simulink model "Quad23"  (R2019a)
settings: Solver=ode4  StartTime=0.0  StopTime=23.06  FixedStep=Ts  RelTol=1e-3
values from neighbouring files (symbols this model uses):
  Am = A-B*K_PP    [ALTITUDE_PLUS_ATTITUDE_CONTROL.m]    (also in ALTITUDE_PLUS_ATTITUDE_CONTROL2.m; ALTITUDE_PLUS_ATTITUDE_CONTROL23.m)
  ATTITUDE0 = 1/60*ones(3,1)    [SETUP.m]    (also in SETUP2.m; SETUP23.m)
  Bm = B    [ALTITUDE_PLUS_ATTITUDE_CONTROL.m]    (also in ALTITUDE_PLUS_ATTITUDE_CONTROL2.m; ALTITUDE_PLUS_ATTITUDE_CONTROL23.m)
  Bum = [1 0 0 ... (first row only)    [ALTITUDE_PLUS_ATTITUDE_CONTROL.m]    (also in ALTITUDE_PLUS_ATTITUDE_CONTROL2.m; ALTITUDE_PLUS_ATTITUDE_CONTROL23.m)
  C = [1 0 0 0 0 0 0 ... (first row only)    [ALTITUDE_PLUS_ATTITUDE_CONTROL.m]    (also in ALTITUDE_PLUS_ATTITUDE_CONTROL2.m; ALTITUDE_PLUS_ATTITUDE_CONTROL23.m; LINEARIZZA_ESTRAI.m = [1 0 0 0 0 0 0 0 0 0 0 0)
  D = 1/s    [ALTITUDE_PLUS_ATTITUDE_CONTROL.m]    (also in ALTITUDE_PLUS_ATTITUDE_CONTROL2.m; ALTITUDE_PLUS_ATTITUDE_CONTROL23.m; LINEARIZZA_ESTRAI.m = [0 0 0 0)
  DEN_TF_eta2m_11 = cell2mat(TF_eta2m.Denominator(1,1))    [ALTITUDE_PLUS_ATTITUDE_CONTROL.m]    (also in ALTITUDE_PLUS_ATTITUDE_CONTROL2.m; ALTITUDE_PLUS_ATTITUDE_CONTROL23.m)
  DEN_TF_eta2m_12 = cell2mat(TF_eta2m.Denominator(1,2))    [ALTITUDE_PLUS_ATTITUDE_CONTROL.m]    (also in ALTITUDE_PLUS_ATTITUDE_CONTROL2.m; ALTITUDE_PLUS_ATTITUDE_CONTROL23.m)
  DEN_TF_eta2m_13 = cell2mat(TF_eta2m.Denominator(1,3))    [ALTITUDE_PLUS_ATTITUDE_CONTROL.m]    (also in ALTITUDE_PLUS_ATTITUDE_CONTROL2.m; ALTITUDE_PLUS_ATTITUDE_CONTROL23.m)
  DEN_TF_eta2m_21 = cell2mat(TF_eta2m.Denominator(2,1))    [ALTITUDE_PLUS_ATTITUDE_CONTROL.m]    (also in ALTITUDE_PLUS_ATTITUDE_CONTROL2.m; ALTITUDE_PLUS_ATTITUDE_CONTROL23.m)
  DEN_TF_eta2m_22 = cell2mat(TF_eta2m.Denominator(2,2))    [ALTITUDE_PLUS_ATTITUDE_CONTROL.m]    (also in ALTITUDE_PLUS_ATTITUDE_CONTROL2.m; ALTITUDE_PLUS_ATTITUDE_CONTROL23.m)
  DEN_TF_eta2m_23 = cell2mat(TF_eta2m.Denominator(2,3))    [ALTITUDE_PLUS_ATTITUDE_CONTROL.m]    (also in ALTITUDE_PLUS_ATTITUDE_CONTROL2.m; ALTITUDE_PLUS_ATTITUDE_CONTROL23.m)
  DEN_TF_eta2m_31 = cell2mat(TF_eta2m.Denominator(3,1))    [ALTITUDE_PLUS_ATTITUDE_CONTROL.m]    (also in ALTITUDE_PLUS_ATTITUDE_CONTROL2.m; ALTITUDE_PLUS_ATTITUDE_CONTROL23.m)
  DEN_TF_eta2m_32 = cell2mat(TF_eta2m.Denominator(3,2))    [ALTITUDE_PLUS_ATTITUDE_CONTROL.m]    (also in ALTITUDE_PLUS_ATTITUDE_CONTROL2.m; ALTITUDE_PLUS_ATTITUDE_CONTROL23.m)
  DEN_TF_eta2m_33 = cell2mat(TF_eta2m.Denominator(3,3))    [ALTITUDE_PLUS_ATTITUDE_CONTROL.m]    (also in ALTITUDE_PLUS_ATTITUDE_CONTROL2.m; ALTITUDE_PLUS_ATTITUDE_CONTROL23.m)
  DEN_TF_eta2m_41 = cell2mat(TF_eta2m.Denominator(4,1))    [ALTITUDE_PLUS_ATTITUDE_CONTROL.m]    (also in ALTITUDE_PLUS_ATTITUDE_CONTROL2.m; ALTITUDE_PLUS_ATTITUDE_CONTROL23.m)
  DEN_TF_eta2m_42 = cell2mat(TF_eta2m.Denominator(4,2))    [ALTITUDE_PLUS_ATTITUDE_CONTROL.m]    (also in ALTITUDE_PLUS_ATTITUDE_CONTROL2.m; ALTITUDE_PLUS_ATTITUDE_CONTROL23.m)
  DEN_TF_eta2m_43 = cell2mat(TF_eta2m.Denominator(4,3))    [ALTITUDE_PLUS_ATTITUDE_CONTROL.m]    (also in ALTITUDE_PLUS_ATTITUDE_CONTROL2.m; ALTITUDE_PLUS_ATTITUDE_CONTROL23.m)
  denD = cell2mat(D.Denominator)    [ALTITUDE_PLUS_ATTITUDE_CONTROL.m]    (also in ALTITUDE_PLUS_ATTITUDE_CONTROL2.m; ALTITUDE_PLUS_ATTITUDE_CONTROL23.m)
  g = 9.81    [SETUP.m]    (also in SETUP2.m; SETUP23.m)
  inertia = diag([Ix,Iy,Iz])    [ALTITUDE_PLUS_ATTITUDE_CONTROL.m]    (also in ALTITUDE_PLUS_ATTITUDE_CONTROL2.m; ALTITUDE_PLUS_ATTITUDE_CONTROL23.m; SETUP.m; SETUP2.m)
  K = 180*eye(m_)    [ALTITUDE_PLUS_ATTITUDE_CONTROL.m]    (also in ALTITUDE_PLUS_ATTITUDE_CONTROL2.m; ALTITUDE_PLUS_ATTITUDE_CONTROL23.m)
  K_PP = place(A,B,pole_TARGET)    [ALTITUDE_PLUS_ATTITUDE_CONTROL.m]    (also in ALTITUDE_PLUS_ATTITUDE_CONTROL2.m; ALTITUDE_PLUS_ATTITUDE_CONTROL23.m)
  Kg = -(C*Am^-1*Bm)^-1    [ALTITUDE_PLUS_ATTITUDE_CONTROL.m]    (also in ALTITUDE_PLUS_ATTITUDE_CONTROL2.m; ALTITUDE_PLUS_ATTITUDE_CONTROL23.m)
  Ksp = -eye(size(Am))*0    [ALTITUDE_PLUS_ATTITUDE_CONTROL.m]    (also in ALTITUDE_PLUS_ATTITUDE_CONTROL2.m; ALTITUDE_PLUS_ATTITUDE_CONTROL23.m)
  LAMBDA = [Kf Kf Kf Kf ... (first row only)    [SETUP.m]    (also in SETUP2.m; SETUP23.m)
  LAMBDA_true = LAMBDA +0.005*randn(size(LAMBDA))*0    [ALTITUDE_PLUS_ATTITUDE_CONTROL.m]    (also in ALTITUDE_PLUS_ATTITUDE_CONTROL2.m; ALTITUDE_PLUS_ATTITUDE_CONTROL23.m)
  m = 2.356    [ALTITUDE_PLUS_ATTITUDE_CONTROL.m]    (also in ALTITUDE_PLUS_ATTITUDE_CONTROL2.m; ALTITUDE_PLUS_ATTITUDE_CONTROL23.m; SETUP.m; SETUP2.m = 0.3)
  n_ = 7    [ALTITUDE_PLUS_ATTITUDE_CONTROL.m]    (also in ALTITUDE_PLUS_ATTITUDE_CONTROL2.m; ALTITUDE_PLUS_ATTITUDE_CONTROL23.m)
  NUM_TF_eta2m_11 = cell2mat(TF_eta2m.Numerator(1,1))    [ALTITUDE_PLUS_ATTITUDE_CONTROL.m]    (also in ALTITUDE_PLUS_ATTITUDE_CONTROL2.m; ALTITUDE_PLUS_ATTITUDE_CONTROL23.m)
  NUM_TF_eta2m_12 = cell2mat(TF_eta2m.Numerator(1,2))    [ALTITUDE_PLUS_ATTITUDE_CONTROL.m]    (also in ALTITUDE_PLUS_ATTITUDE_CONTROL2.m; ALTITUDE_PLUS_ATTITUDE_CONTROL23.m)
  NUM_TF_eta2m_13 = cell2mat(TF_eta2m.Numerator(1,3))    [ALTITUDE_PLUS_ATTITUDE_CONTROL.m]    (also in ALTITUDE_PLUS_ATTITUDE_CONTROL2.m; ALTITUDE_PLUS_ATTITUDE_CONTROL23.m)
  NUM_TF_eta2m_21 = cell2mat(TF_eta2m.Numerator(2,1))    [ALTITUDE_PLUS_ATTITUDE_CONTROL.m]    (also in ALTITUDE_PLUS_ATTITUDE_CONTROL2.m; ALTITUDE_PLUS_ATTITUDE_CONTROL23.m)
  NUM_TF_eta2m_22 = cell2mat(TF_eta2m.Numerator(2,2))    [ALTITUDE_PLUS_ATTITUDE_CONTROL.m]    (also in ALTITUDE_PLUS_ATTITUDE_CONTROL2.m; ALTITUDE_PLUS_ATTITUDE_CONTROL23.m)
  NUM_TF_eta2m_23 = cell2mat(TF_eta2m.Numerator(2,3))    [ALTITUDE_PLUS_ATTITUDE_CONTROL.m]    (also in ALTITUDE_PLUS_ATTITUDE_CONTROL2.m; ALTITUDE_PLUS_ATTITUDE_CONTROL23.m)
  NUM_TF_eta2m_31 = cell2mat(TF_eta2m.Numerator(3,1))    [ALTITUDE_PLUS_ATTITUDE_CONTROL.m]    (also in ALTITUDE_PLUS_ATTITUDE_CONTROL2.m; ALTITUDE_PLUS_ATTITUDE_CONTROL23.m)
  NUM_TF_eta2m_32 = cell2mat(TF_eta2m.Numerator(3,2))    [ALTITUDE_PLUS_ATTITUDE_CONTROL.m]    (also in ALTITUDE_PLUS_ATTITUDE_CONTROL2.m; ALTITUDE_PLUS_ATTITUDE_CONTROL23.m)
  NUM_TF_eta2m_33 = cell2mat(TF_eta2m.Numerator(3,3))    [ALTITUDE_PLUS_ATTITUDE_CONTROL.m]    (also in ALTITUDE_PLUS_ATTITUDE_CONTROL2.m; ALTITUDE_PLUS_ATTITUDE_CONTROL23.m)
  NUM_TF_eta2m_41 = cell2mat(TF_eta2m.Numerator(4,1))    [ALTITUDE_PLUS_ATTITUDE_CONTROL.m]    (also in ALTITUDE_PLUS_ATTITUDE_CONTROL2.m; ALTITUDE_PLUS_ATTITUDE_CONTROL23.m)
  NUM_TF_eta2m_42 = cell2mat(TF_eta2m.Numerator(4,2))    [ALTITUDE_PLUS_ATTITUDE_CONTROL.m]    (also in ALTITUDE_PLUS_ATTITUDE_CONTROL2.m; ALTITUDE_PLUS_ATTITUDE_CONTROL23.m)
  NUM_TF_eta2m_43 = cell2mat(TF_eta2m.Numerator(4,3))    [ALTITUDE_PLUS_ATTITUDE_CONTROL.m]    (also in ALTITUDE_PLUS_ATTITUDE_CONTROL2.m; ALTITUDE_PLUS_ATTITUDE_CONTROL23.m)
  numD = cell2mat(D.Numerator)    [ALTITUDE_PLUS_ATTITUDE_CONTROL.m]    (also in ALTITUDE_PLUS_ATTITUDE_CONTROL2.m; ALTITUDE_PLUS_ATTITUDE_CONTROL23.m)
  omega0 = eye(m_)    [ALTITUDE_PLUS_ATTITUDE_CONTROL.m]    (also in ALTITUDE_PLUS_ATTITUDE_CONTROL2.m; ALTITUDE_PLUS_ATTITUDE_CONTROL23.m)
  omega_start = 0*ones(3,1)    [SETUP.m]    (also in SETUP2.m; SETUP23.m)
  phi_ref = 0/60    (= 0)    [SETUP.m]    (also in SETUP2.m = attitude(:,2); SETUP23.m = attitude(:,2))
  POS0 = 0*ones(3,1)    [SETUP.m]    (also in SETUP2.m; SETUP23.m)
  psi_ref = 0/60    (= 0)    [SETUP.m]    (also in SETUP2.m = attitude(:,3); SETUP23.m = attitude(:,3))
  theta_ref = 0/60    (= 0)    [SETUP.m]    (also in SETUP2.m = attitude(:,1); SETUP23.m = attitude(:,1))
  Ts = 0.01    [ALTITUDE_PLUS_ATTITUDE_CONTROL.m]    (also in ALTITUDE_PLUS_ATTITUDE_CONTROL2.m; ALTITUDE_PLUS_ATTITUDE_CONTROL23.m)
  V0 = 0*ones(3,1)    [SETUP.m]    (also in SETUP2.m; SETUP23.m)
undefined symbols (not defined in the file or in its folder): magnitude
libraries: simulink x6, vrlib x2, dspinverses x1, dspmtrx3 x1
settings Model: Creator=Paolo  LastModifiedBy=sushant
settings DataIOCC: ReturnWorkspaceOutputs=off
settings DebuggingCC: ArithmeticOperatorsInVariantConditions=warning
settings SFSimCC: SimUseLocalCustomCode=off
settings RTWCC: RTWUseLocalCustomCode=off
settings CodeAppCC: StateflowObjectComments=on

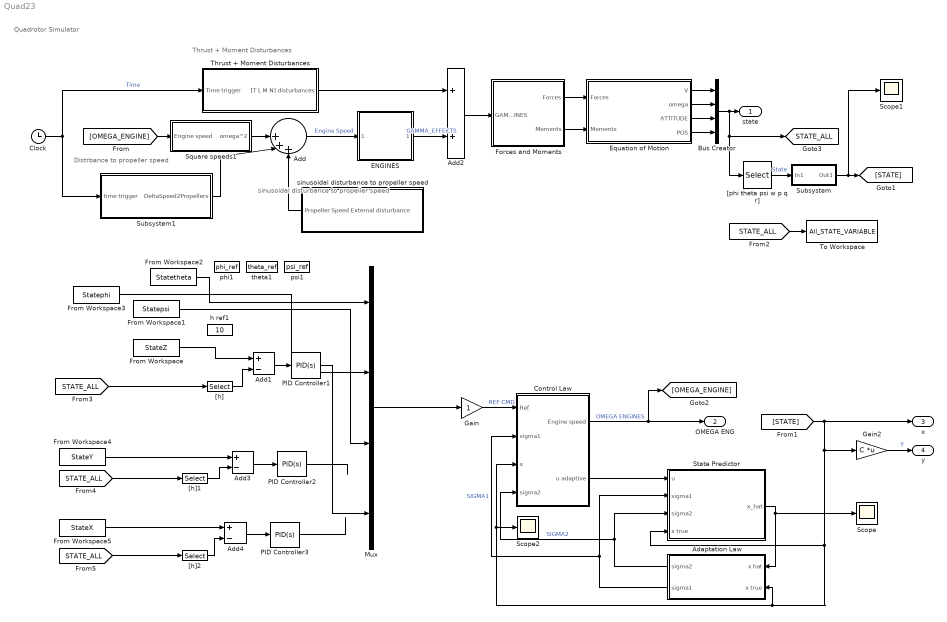
== system Quad23 ==
  note: sinusoidal disturbance to propeller speed
  note: Distrbance to
      | propeller
      | speed
  note: Thrust + Moment
      | Disturbances
  note: Quadrotor Simulator
  Adaptation Law : Subsystem  mask{Am=Am, B=[Bm Bum], Ts=Ts}
      mask prompts: Am "Enter desired dynamic matrix"; B "Enter B matrix [Bm Bum]"; Ts "Insert time step"
  Add : Sum  Inputs=||+++
  Add1 : Sum  Inputs=+-
  Add2 : Sum
  Add3 : Sum  Inputs=+-
  Add4 : Sum  Inputs=+-
  Bus Creator : BusCreator  Inputs=4
  Clock : Clock
  Control Law : Subsystem
  ENGINES : Subsystem  mask{LAMBDA=LAMBDA_true}
      mask prompts: LAMBDA "Insert Lambda Matrix"
      mask Display: image('g4165.png');
  Equation of Motion : Subsystem  mask{V0=V0, omega0=omega0, ATTITUDE0=ATTITUDE0, POS0=POS0, m=m, inertia=inertia, inertia_inv=inv(inertia)}
      mask prompts: V0 "Insert initial speed (body)"; omega0 "Insert initial rotational speed"; ATTITUDE0 "Insert initial attitude"; POS0 "Insert initial position"; m "Insert mass"; inertia "Insert inertia matrix"; inertia_inv "Insert inverse inertia matrix"
      mask DialogControl DescGroupVar Prompt: Insert parameters
      mask DialogControl DescTextVar Prompt: The parameters neeeded for the equation of motion
      mask Display: image('512px-Quadrotorhover.svg.png');
  Forces and Moments : Subsystem
  From Workspace : FromWorkspace  VariableName=StateZ  OutDataTypeStr=double  SampleTime=0.01
  From Workspace1 : FromWorkspace  VariableName=Statepsi  OutDataTypeStr=double  SampleTime=0.01
  From Workspace2 : FromWorkspace  VariableName=Statetheta  OutDataTypeStr=double  SampleTime=0.01
  From Workspace3 : FromWorkspace  VariableName=Statephi  OutDataTypeStr=double  SampleTime=0.01
  From Workspace4 : FromWorkspace  VariableName=StateY  OutDataTypeStr=double  SampleTime=0.02
  From Workspace5 : FromWorkspace  VariableName=StateX  OutDataTypeStr=double  SampleTime=0.02
  Gain : Gain
  Gain2 : Gain  Gain=C  Multiplication=Matrix(K*u)
  Mux : Mux
  PID Controller1 : simulink/Continuous/PID Controller  Controller=PID  Form=Parallel  TimeDomain=Continuous-time  SampleTime=-1  IntegratorMethod=Forward Euler  FilterMethod=Forward Euler  ControllerParametersSource=internal  P=6.60433562014458  I=3.10197576305367/2  D=1.82120992541133  UseFilter=on  N=200  TunerSelectOption=Transfer Function Based (PID Tuner App)  InitialConditionSource=internal  InitialConditionForIntegrator=0  InitialConditionForFilter=0  DifferentiatorICPrevScaledInput=0  ExternalReset=none  TrackingMode=off  Kt=1  LimitOutput=on  UpperSaturationLimit=1  LowerSaturationLimit=-1  LinearizeAsGain=on  AntiWindupMode=back-calculation  Kb=1  POutMin=[]  POutMax=[]  IOutMin=[]  IOutMax=[]  DOutMin=[]  DOutMax=[]  NOutMin=[]  NOutMax=[]  SumOutMin=[]  SumOutMax=[]  SaturationOutMin=[]  SaturationOutMax=[]  PParamMin=[]  PParamMax=[]  IParamMin=[]  IParamMax=[]  DParamMin=[]  DParamMax=[]  NParamMin=[]  NParamMax=[]  KbParamMin=[]  KbParamMax=[]  KtParamMin=[]  KtParamMax=[]  KbOutMin=[]  KbOutMax=[]  KtOutMin=[]  KtOutMax=[]  IntegratorOutMin=[]  IntegratorOutMax=[]  FilterOutMin=[]  FilterOutMax=[]  SumI1OutMin=[]  SumI1OutMax=[]  SumI2OutMin=[]  SumI2OutMax=[]  SumI3OutMin=[]  SumI3OutMax=[]  SumI4OutMin=[]  SumI4OutMax=[]  SumDOutMin=[]  SumDOutMax=[]  DifferentiatorOutMin=[]  DifferentiatorOutMax=[]  FilterDiffOutCoefMin=[]  FilterDiffOutCoefMax=[]  ReciprocalOutMin=[]  ReciprocalOutMax=[]  SumDenOutMin=[]  SumDenOutMax=[]  SumNumOutMin=[]  SumNumOutMax=[]  DivideOutMin=[]  DivideOutMax=[]  IntegratorContinuousStateAttributes=''  IntegratorStateMustResolveToSignalObject=off  IntegratorRTWStateStorageClass=Auto  FilterContinuousStateAttributes=''  FilterStateMustResolveToSignalObject=off  FilterRTWStateStorageClass=Auto  ParallelPVariant=InternalParameters  IdealPVariant=Disabled  IVariant=InternalParameters  DVariant=InternalParameters  IntegratorVariant=Continuous  SatVariant=Enabled  AWVariant=BackCalculation  PCopyVariant=Disabled  TRVariant=Disabled  FdbkBlocksVariant=Forward  IdealPFdbkVariant=Disabled  SatFdbkVariant=Disabled  DerivativeFilterVariant=ContFilter  NVariant=InternalParameters  NCopyVariant=Disabled  FilterICVariant=InternalICsFilter  IntegratorICVariant=InternalICs  ExternalResetVariant=Disabled  TRSumVariant=Passthrough  SumFdbkVariant=Disabled  SumVariant=Sum_PID
  PID Controller2 : simulink/Continuous/PID Controller  Controller=PID  Form=Parallel  TimeDomain=Continuous-time  SampleTime=-1  IntegratorMethod=Forward Euler  FilterMethod=Forward Euler  ControllerParametersSource=internal  P=6.60433562014458  I=3.10197576305367/2  D=1.82120992541133  UseFilter=on  N=200  TunerSelectOption=Transfer Function Based (PID Tuner App)  InitialConditionSource=internal  InitialConditionForIntegrator=0  InitialConditionForFilter=0  DifferentiatorICPrevScaledInput=0  ExternalReset=none  TrackingMode=off  Kt=1  LimitOutput=on  UpperSaturationLimit=1  LowerSaturationLimit=-1  LinearizeAsGain=on  AntiWindupMode=back-calculation  Kb=1  POutMin=[]  POutMax=[]  IOutMin=[]  IOutMax=[]  DOutMin=[]  DOutMax=[]  NOutMin=[]  NOutMax=[]  SumOutMin=[]  SumOutMax=[]  SaturationOutMin=[]  SaturationOutMax=[]  PParamMin=[]  PParamMax=[]  IParamMin=[]  IParamMax=[]  DParamMin=[]  DParamMax=[]  NParamMin=[]  NParamMax=[]  KbParamMin=[]  KbParamMax=[]  KtParamMin=[]  KtParamMax=[]  KbOutMin=[]  KbOutMax=[]  KtOutMin=[]  KtOutMax=[]  IntegratorOutMin=[]  IntegratorOutMax=[]  FilterOutMin=[]  FilterOutMax=[]  SumI1OutMin=[]  SumI1OutMax=[]  SumI2OutMin=[]  SumI2OutMax=[]  SumI3OutMin=[]  SumI3OutMax=[]  SumI4OutMin=[]  SumI4OutMax=[]  SumDOutMin=[]  SumDOutMax=[]  DifferentiatorOutMin=[]  DifferentiatorOutMax=[]  FilterDiffOutCoefMin=[]  FilterDiffOutCoefMax=[]  ReciprocalOutMin=[]  ReciprocalOutMax=[]  SumDenOutMin=[]  SumDenOutMax=[]  SumNumOutMin=[]  SumNumOutMax=[]  DivideOutMin=[]  DivideOutMax=[]  IntegratorContinuousStateAttributes=''  IntegratorStateMustResolveToSignalObject=off  IntegratorRTWStateStorageClass=Auto  FilterContinuousStateAttributes=''  FilterStateMustResolveToSignalObject=off  FilterRTWStateStorageClass=Auto  ParallelPVariant=InternalParameters  IdealPVariant=Disabled  IVariant=InternalParameters  DVariant=InternalParameters  IntegratorVariant=Continuous  SatVariant=Enabled  AWVariant=BackCalculation  PCopyVariant=Disabled  TRVariant=Disabled  FdbkBlocksVariant=Forward  IdealPFdbkVariant=Disabled  SatFdbkVariant=Disabled  DerivativeFilterVariant=ContFilter  NVariant=InternalParameters  NCopyVariant=Disabled  FilterICVariant=InternalICsFilter  IntegratorICVariant=InternalICs  ExternalResetVariant=Disabled  TRSumVariant=Passthrough  SumFdbkVariant=Disabled  SumVariant=Sum_PID
  PID Controller3 : simulink/Continuous/PID Controller  Controller=PID  Form=Parallel  TimeDomain=Continuous-time  SampleTime=-1  IntegratorMethod=Forward Euler  FilterMethod=Forward Euler  ControllerParametersSource=internal  P=6.60433562014458  I=3.10197576305367/2  D=1.82120992541133  UseFilter=on  N=200  TunerSelectOption=Transfer Function Based (PID Tuner App)  InitialConditionSource=internal  InitialConditionForIntegrator=0  InitialConditionForFilter=0  DifferentiatorICPrevScaledInput=0  ExternalReset=none  TrackingMode=off  Kt=1  LimitOutput=on  UpperSaturationLimit=1  LowerSaturationLimit=-1  LinearizeAsGain=on  AntiWindupMode=back-calculation  Kb=1  POutMin=[]  POutMax=[]  IOutMin=[]  IOutMax=[]  DOutMin=[]  DOutMax=[]  NOutMin=[]  NOutMax=[]  SumOutMin=[]  SumOutMax=[]  SaturationOutMin=[]  SaturationOutMax=[]  PParamMin=[]  PParamMax=[]  IParamMin=[]  IParamMax=[]  DParamMin=[]  DParamMax=[]  NParamMin=[]  NParamMax=[]  KbParamMin=[]  KbParamMax=[]  KtParamMin=[]  KtParamMax=[]  KbOutMin=[]  KbOutMax=[]  KtOutMin=[]  KtOutMax=[]  IntegratorOutMin=[]  IntegratorOutMax=[]  FilterOutMin=[]  FilterOutMax=[]  SumI1OutMin=[]  SumI1OutMax=[]  SumI2OutMin=[]  SumI2OutMax=[]  SumI3OutMin=[]  SumI3OutMax=[]  SumI4OutMin=[]  SumI4OutMax=[]  SumDOutMin=[]  SumDOutMax=[]  DifferentiatorOutMin=[]  DifferentiatorOutMax=[]  FilterDiffOutCoefMin=[]  FilterDiffOutCoefMax=[]  ReciprocalOutMin=[]  ReciprocalOutMax=[]  SumDenOutMin=[]  SumDenOutMax=[]  SumNumOutMin=[]  SumNumOutMax=[]  DivideOutMin=[]  DivideOutMax=[]  IntegratorContinuousStateAttributes=''  IntegratorStateMustResolveToSignalObject=off  IntegratorRTWStateStorageClass=Auto  FilterContinuousStateAttributes=''  FilterStateMustResolveToSignalObject=off  FilterRTWStateStorageClass=Auto  ParallelPVariant=InternalParameters  IdealPVariant=Disabled  IVariant=InternalParameters  DVariant=InternalParameters  IntegratorVariant=Continuous  SatVariant=Enabled  AWVariant=BackCalculation  PCopyVariant=Disabled  TRVariant=Disabled  FdbkBlocksVariant=Forward  IdealPFdbkVariant=Disabled  SatFdbkVariant=Disabled  DerivativeFilterVariant=ContFilter  NVariant=InternalParameters  NCopyVariant=Disabled  FilterICVariant=InternalICsFilter  IntegratorICVariant=InternalICs  ExternalResetVariant=Disabled  TRSumVariant=Passthrough  SumFdbkVariant=Disabled  SumVariant=Sum_PID
  Scope : Scope
  Scope1 : Scope
  Scope2 : Scope
  Square speeds1 : Subsystem
  State Predictor : Subsystem  mask{Am=Am, Bm=Bm, Bum=Bum, Ksp=Ksp, x0hat=zeros(n_,1), omega0=eye(4)}
      mask prompts: Am "Enter desired dynamic matrix"; Bm "Enter matched control matrix"; Bum "Enter unmatched control matrix"; Ksp "Enter estimator matrix"; x0hat "Enter initial condition"; omega0 "Enter control disturbances"
  Subsystem : Subsystem
  Subsystem1 : Subsystem
  Thrust + Moment Disturbances : Subsystem
  To Workspace : ToWorkspace  VariableName=All_STATE_VARIABLE  SaveFormat=Timeseries  SampleTime=-1
  "[h]" : Selector  InputPortWidth=12  IndexOptions=Index vector (dialog)  Indices=[12]  OutputSizes=1
  "[h]1" : Selector  InputPortWidth=12  IndexOptions=Index vector (dialog)  Indices=[11]  OutputSizes=1
  "[h]2" : Selector  InputPortWidth=12  IndexOptions=Index vector (dialog)  Indices=[10]  OutputSizes=1
  "[phi theta psi w p q r]" : Selector  InputPortWidth=12  IndexOptions=Index vector (dialog)  Indices=[7 8 9 3 4 5 6]  OutputSizes=1
  h ref1 : Constant  Value=10
  phi1 : Constant  Value=phi_ref
  psi1 : Constant  Value=psi_ref
  sinusoidal disturbance to propeller speed : Subsystem
  theta1 : Constant  Value=theta_ref
  state : Outport
  OMEGA ENG : Outport  Port=2
  x : Outport  Port=3
  y : Outport  Port=4
  tag scope: STATE_ALL=global
  wires:
  Equation of Motion/3(ATTITUDE) -> Bus Creator/3
  Equation of Motion/4(POS) -> Bus Creator/4
  Bus Creator/1 -> [STATE_ALL], "[phi theta psi w p q r]"/1, state/1
  Equation of Motion/1(V) -> Bus Creator/1
  Equation of Motion/2(omega) -> Bus Creator/2
  Forces and Moments/1(Forces) -> Equation of Motion/1(Forces)
  Forces and Moments/2(Moments) -> Equation of Motion/2(Moments)
  State Predictor/1(x_hat) -> Adaptation Law/1(x hat), Scope/1
  Adaptation Law/1(sigma2) -> State Predictor/3(sigma2), Control Law/4(sigma2)  "SIGMA2"
  Adaptation Law/2(sigma1) -> Control Law/2(sigma1), State Predictor/2(sigma1)  "SIGMA1"
  Mux/1 -> Gain/1
  Gain/1 -> Control Law/1(Ref)  "REF CMD"
  "[phi theta psi w p q r]"/1 -> Subsystem/1(In1)  "State"
  Gain2/1 -> y/1  "Y"
  ENGINES/1(GAMMA EFFECTS) -> Add2/2  "GAMMA_EFFECTS"
  Control Law/2(u adaptive) -> State Predictor/1(u)
  Add/1 -> ENGINES/1(OMEGA  SQUARE)  "Engine Speed"
  Clock/1 -> Subsystem1/1(time trigger), Thrust + Moment Disturbances/1(Time trigger)  "Time"
  Add2/1 -> Forces and Moments/1(GAMMA ENGINES)
  [OMEGA_ENGINE] -> Square speeds1/1(Engine speed)
  Square speeds1/1(omega^2) -> Add/1
  [STATE] -> Gain2/1, Scope2/1, Control Law/3(x), Adaptation Law/2(x true), State Predictor/4(x true), x/1
  Control Law/1(Engine speed) -> [OMEGA_ENGINE], OMEGA ENG/1  "OMEGA ENGINES"
  Subsystem/1(Out1) -> Scope1/1, [STATE]
  PID Controller1/1 -> Mux/4
  From Workspace1/1 -> Mux/3
  From Workspace3/1 -> Mux/2
  From Workspace2/1 -> Mux/1
  [STATE_ALL] -> To Workspace/1
  [STATE_ALL] -> "[h]"/1
  Add1/1 -> PID Controller1/1
  "[h]"/1 -> Add1/2
  From Workspace/1 -> Add1/1
  Thrust + Moment Disturbances/1("[T L M N] disturbances") -> Add2/1
  Subsystem1/1(DeltaSpeed2Propellers) -> Add/2
  sinusoidal disturbance to propeller speed/1(Propeller Speed External disturbance) -> Add/3
  From Workspace4/1 -> Add3/1
  "[h]1"/1 -> Add3/2
  Add3/1 -> PID Controller2/1
  [STATE_ALL] -> "[h]1"/1
  [STATE_ALL] -> "[h]2"/1
  Add4/1 -> PID Controller3/1
  "[h]2"/1 -> Add4/2
  From Workspace5/1 -> Add4/1
  PID Controller3/1 -> ?
  PID Controller2/1 -> ?

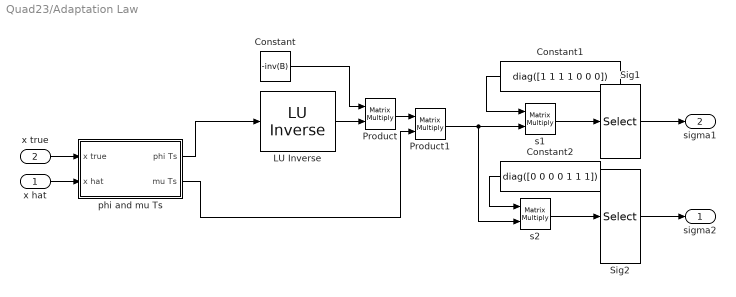
== system Quad23/Adaptation Law ==
  x hat : Inport
  x true : Inport  Port=2
  " LU Inverse" : dspinverses/ LU Inverse
      settings: SourceProductName=DSP System Toolbox
  Constant : Constant  Value=-inv(B)
  Constant1 : Constant  Value=diag([1 1 1 1 0 0 0])
  Constant2 : Constant  Value=diag([0 0 0 0 1 1 1])
  Product : Product  Multiplication=Matrix(*)
  Product1 : Product  Multiplication=Matrix(*)
  Sig1 : Selector  InputPortWidth=7  IndexOptions=Index vector (dialog)  Indices=[1 2 3 4]  OutputSizes=1
  Sig2 : Selector  InputPortWidth=7  IndexOptions=Index vector (dialog)  Indices=[5 6 7]  OutputSizes=1
  phi and mu Ts : Subsystem
  s1 : Product  Multiplication=Matrix(*)
  s2 : Product  Multiplication=Matrix(*)
  sigma2 : Outport
  sigma1 : Outport  Port=2
  wires:
  Sig2/1 -> sigma2/1
  Sig1/1 -> sigma1/1
  Constant2/1 -> s2/1
  Constant1/1 -> s1/1
  s1/1 -> Sig1/1
  x true/1 -> phi and mu Ts/1(x true)
  x hat/1 -> phi and mu Ts/2(x hat)
  phi and mu Ts/1(phi Ts) -> " LU Inverse"/1
  phi and mu Ts/2(mu Ts) -> Product1/2
  " LU Inverse"/1 -> Product/2
  Constant/1 -> Product/1
  Product1/1 -> s1/2, s2/2
  Product/1 -> Product1/1
  s2/1 -> Sig2/1

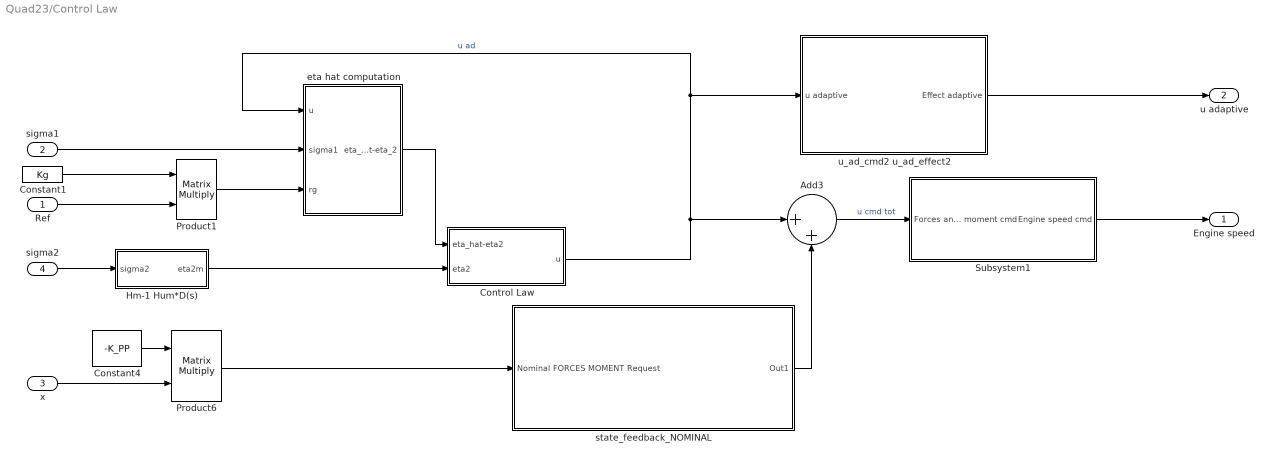
== system Quad23/Control Law ==
  Ref : Inport
  sigma1 : Inport  Port=2
  x : Inport  Port=3
  sigma2 : Inport  Port=4
  Add3 : Sum  Inputs=|++
  Constant1 : Constant  Value=Kg
  Constant4 : Constant  Value=-K_PP
  Control Law : Subsystem
  Hm-1 Hum*D(s) : Subsystem
  Product1 : Product  Multiplication=Matrix(*)  RndMeth=Zero
  Product6 : Product  Multiplication=Matrix(*)  RndMeth=Zero
  Subsystem1 : Subsystem
  eta hat computation : Subsystem
  state_feedback_NOMINAL : Subsystem
  u_ad_cmd2 u_ad_effect2 : Subsystem
  Engine speed : Outport
  u adaptive : Outport  Port=2
  wires:
  Constant1/1 -> Product1/1
  Ref/1 -> Product1/2
  Add3/1 -> Subsystem1/1(Forces and moment cmd)  "u cmd tot"
  x/1 -> Product6/2
  Constant4/1 -> Product6/1
  Control Law/1(u) -> Add3/1, u_ad_cmd2 u_ad_effect2/1(u adaptive), eta hat computation/1(u)  "u ad"
  sigma1/1 -> eta hat computation/2(sigma1)
  Product1/1 -> eta hat computation/3(rg)
  Hm-1 Hum*D(s)/1(eta2m) -> Control Law/2(eta2)
  eta hat computation/1(eta_hat-eta_2) -> Control Law/1(eta_hat-eta2)
  sigma2/1 -> Hm-1 Hum*D(s)/1(sigma2)
  Subsystem1/1(Engine speed cmd) -> Engine speed/1
  Product6/1 -> state_feedback_NOMINAL/1(Nominal FORCES MOMENT Request)
  u_ad_cmd2 u_ad_effect2/1(Effect adaptive) -> u adaptive/1
  state_feedback_NOMINAL/1(Out1) -> Add3/2

== system Quad23/ENGINES ==
  OMEGA  SQUARE : Inport
  Constant : Constant  Value=LAMBDA
  Product : Product  Multiplication=Matrix(*)
  GAMMA EFFECTS : Outport
  wires:
  Constant/1 -> Product/1
  Product/1 -> GAMMA EFFECTS/1
  OMEGA  SQUARE/1 -> Product/2

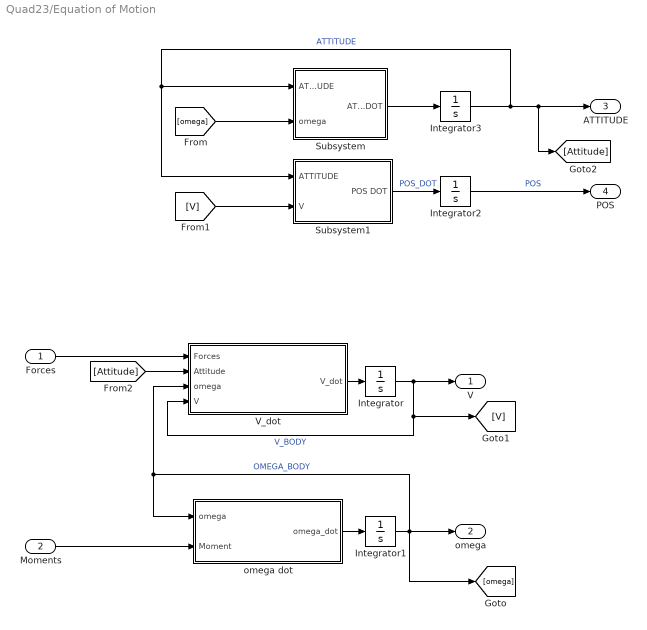
== system Quad23/Equation of Motion ==
  Forces : Inport
  Moments : Inport  Port=2
  Integrator : Integrator  InitialCondition=V0
  Integrator1 : Integrator  InitialCondition=omega_start
  Integrator2 : Integrator  InitialCondition=POS0
  Integrator3 : Integrator  InitialCondition=ATTITUDE0
  Subsystem : Subsystem
  Subsystem1 : Subsystem
  "V_dot " : Subsystem
  omega dot : Subsystem
  V : Outport
  omega : Outport  Port=2
  ATTITUDE : Outport  Port=3
  POS : Outport  Port=4
  wires:
  omega dot/1(omega_dot) -> Integrator1/1
  Integrator1/1 -> omega/1, [omega], omega dot/1(omega), "V_dot "/3(omega)  "OMEGA_BODY"
  "V_dot "/1(V_dot) -> Integrator/1
  Subsystem/1(ATTITUDE DOT) -> Integrator3/1
  [omega] -> Subsystem/2(omega)
  Integrator/1 -> V/1, [V], "V_dot "/4(V)  "V_BODY"
  Subsystem1/1(POS DOT) -> Integrator2/1  "POS_DOT"
  Integrator3/1 -> [Attitude], ATTITUDE/1, Subsystem1/1(ATTITUDE), Subsystem/1(ATTITUDE)  "ATTITUDE"
  Integrator2/1 -> POS/1  "POS"
  [V] -> Subsystem1/2(V)
  Moments/1 -> omega dot/2(Moment)
  Forces/1 -> "V_dot "/1(Forces)
  [Attitude] -> "V_dot "/2(Attitude)

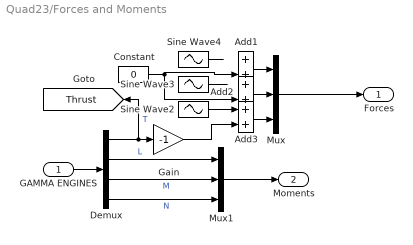
== system Quad23/Forces and Moments ==
  GAMMA ENGINES : Inport
  Add1 : Sum
  Add2 : Sum
  Add3 : Sum
  Constant : Constant  Value=0
  Demux : Demux
  Gain : Gain  Gain=-1
  Mux : Mux  Inputs=3
  Mux1 : Mux  Inputs=3
  Sine Wave2 : Sin  Amplitude=2  Frequency=0.2  SampleTime=0
  Sine Wave3 : Sin  Amplitude=2  Frequency=0.01  Phase=0.4  SampleTime=0
  Sine Wave4 : Sin  Amplitude=0.3  Frequency=0.1  Phase=0.2  SampleTime=0
  Forces : Outport
  Moments : Outport  Port=2
  tag scope: Thrust=global
  wires:
  Mux1/1 -> Moments/1
  GAMMA ENGINES/1 -> Demux/1
  Constant/1 -> Add1/2, Add2/2
  Gain/1 -> Add3/2
  Mux/1 -> Forces/1
  Demux/1 -> [Thrust], Gain/1  "T"
  Demux/3 -> Mux1/2  "M"
  Demux/2 -> Mux1/1  "L"
  Demux/4 -> Mux1/3  "N"
  Add1/1 -> Mux/1
  Add2/1 -> Mux/2
  Add3/1 -> Mux/3
  Sine Wave4/1 -> ?
  Sine Wave3/1 -> ?
  Sine Wave2/1 -> Add3/1

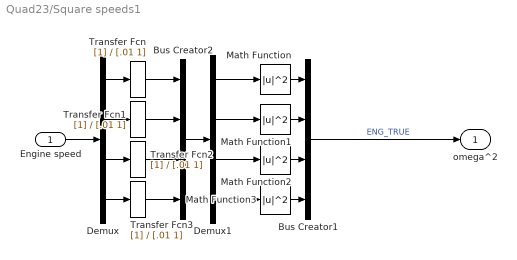
== system Quad23/Square speeds1 ==
  Engine speed : Inport
  Bus Creator1 : BusCreator  Inputs=4
  Bus Creator2 : BusCreator  Inputs=4
  Demux : Demux
  Demux1 : Demux
  Math Function{,1..3} (4 alike) : Math  Operator=magnitude^2  OutputSignalType=real  SaturateOnIntegerOverflow=on
  Transfer Fcn{,1..3} (4 alike) : TransferFcn  Denominator=[.01 1]
  omega^2 : Outport
  wires:
  Bus Creator1/1 -> omega^2/1  "ENG_TRUE"
  Transfer Fcn3/1 -> Bus Creator2/4
  Transfer Fcn2/1 -> Bus Creator2/3
  Transfer Fcn1/1 -> Bus Creator2/2
  Transfer Fcn/1 -> Bus Creator2/1
  Demux/1 -> Transfer Fcn/1
  Math Function/1 -> Bus Creator1/1
  Math Function1/1 -> Bus Creator1/2
  Math Function2/1 -> Bus Creator1/3
  Math Function3/1 -> Bus Creator1/4
  Demux/3 -> Transfer Fcn2/1
  Engine speed/1 -> Demux/1
  Demux/2 -> Transfer Fcn1/1
  Demux/4 -> Transfer Fcn3/1
  Bus Creator2/1 -> Demux1/1
  Demux1/2 -> Math Function1/1
  Demux1/1 -> Math Function/1
  Demux1/3 -> Math Function2/1
  Demux1/4 -> Math Function3/1

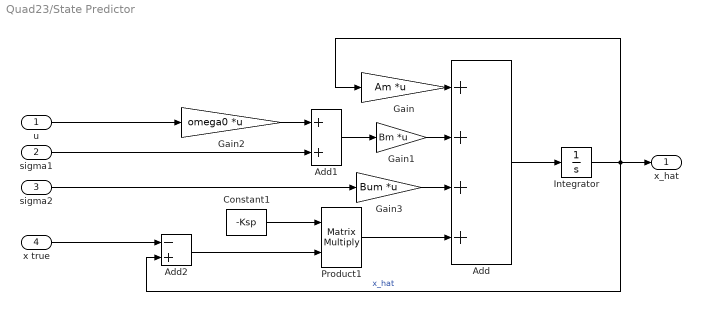
== system Quad23/State Predictor ==
  u : Inport
  sigma1 : Inport  Port=2
  sigma2 : Inport  Port=3
  x true : Inport  Port=4
  Add : Sum  Inputs=++++
  Add1 : Sum
  Add2 : Sum  Inputs=-+
  Constant1 : Constant  Value=-Ksp
  Gain : Gain  Gain=Am  Multiplication=Matrix(K*u)
  Gain1 : Gain  Gain=Bm  Multiplication=Matrix(K*u)
  Gain2 : Gain  Gain=omega0  Multiplication=Matrix(K*u)
  Gain3 : Gain  Gain=Bum  Multiplication=Matrix(K*u)
  Integrator : Integrator  InitialCondition=x0hat
  Product1 : Product  Multiplication=Matrix(*)  RndMeth=Zero
  x_hat : Outport
  wires:
  Integrator/1 -> x_hat/1, Add2/2, Gain/1  "x_hat"
  Add1/1 -> Gain1/1
  Gain3/1 -> Add/3
  Gain1/1 -> Add/2
  Product1/1 -> Add/4
  Gain/1 -> Add/1
  Gain2/1 -> Add1/1
  Add/1 -> Integrator/1
  u/1 -> Gain2/1
  sigma1/1 -> Add1/2
  sigma2/1 -> Gain3/1
  x true/1 -> Add2/1
  Constant1/1 -> Product1/1
  Add2/1 -> Product1/2

== system Quad23/Subsystem ==
  In1 : Inport
  Demux : Demux  Outputs=7
  Gain9 : Gain  Gain=0
  Mux3 : Mux  Inputs=7
  Out1 : Outport
  wires:
  Demux/1 -> Mux3/1
  Demux/3 -> Mux3/3
  Demux/5 -> Mux3/5
  Demux/6 -> Mux3/6
  Demux/2 -> Mux3/2
  Demux/4 -> Gain9/1
  Demux/7 -> Mux3/7
  Gain9/1 -> Mux3/4
  In1/1 -> Demux/1
  Mux3/1 -> Out1/1

== system Quad23/Subsystem1 ==
  time trigger : Inport
  Constant6 : Constant  Value=-[.5 1 2 7]*3
  Constant7 : Constant  Value=-[.5 1 2 7]*0
  Switch : Switch  Criteria=u2 > Threshold  Threshold=20
  DeltaSpeed2Propellers : Outport
  wires:
  Switch/1 -> DeltaSpeed2Propellers/1
  Constant6/1 -> Switch/1
  Constant7/1 -> Switch/3
  time trigger/1 -> Switch/2

== system Quad23/Thrust + Moment Disturbances ==
  Time trigger : Inport
  Constant10 : Constant  Value=-[5 5 -4 .8]*.5
  Constant9 : Constant  Value=-[5 5*0 -2 .8*0]
  Switch1 : Switch  Criteria=u2 > Threshold  Threshold=60
  "[T L M N] disturbances" : Outport
  wires:
  Time trigger/1 -> Switch1/2
  Constant10/1 -> Switch1/1
  Switch1/1 -> "[T L M N] disturbances"/1
  Constant9/1 -> Switch1/3

== system Quad23/sinusoidal disturbance to propeller speed ==
  Mux1 : Mux
  Sine Wave1 : Sin  Amplitude=10  Frequency=10  Phase=-0.5  SampleTime=0
  Sine Wave2 : Sin  Amplitude=8  Frequency=10  SampleTime=0
  Sine Wave3 : Sin  Amplitude=12  Frequency=10  Phase=0.4  SampleTime=0
  Sine Wave4 : Sin  Amplitude=8  Bias=2  Frequency=8  Phase=0.2  SampleTime=0
  Propeller Speed External disturbance : Outport
  wires:
  Sine Wave4/1 -> Mux1/2
  Sine Wave1/1 -> Mux1/1
  Mux1/1 -> Propeller Speed External disturbance/1
  Sine Wave2/1 -> Mux1/4
  Sine Wave3/1 -> Mux1/3

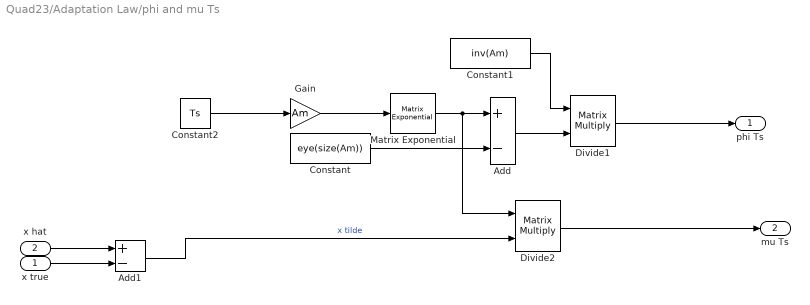
== system Quad23/Adaptation Law/phi and mu Ts ==
  x true : Inport
  x hat : Inport  Port=2
  Add : Sum  Inputs=+-
  Add1 : Sum  Inputs=+-
  Constant : Constant  Value=eye(size(Am))
  Constant1 : Constant  Value=inv(Am)
  Constant2 : Constant  Value=Ts
  Divide1 : Product  Inputs=**  Multiplication=Matrix(*)
  Divide2 : Product  Inputs=**  Multiplication=Matrix(*)
  Gain : Gain  Gain=Am
  Matrix Exponential : dspmtrx3/Matrix Exponential
      settings: SourceProductName=DSP System Toolbox  SourceProductBaseCode=DS
  phi Ts : Outport
  mu Ts : Outport  Port=2
  wires:
  Constant1/1 -> Divide1/1
  Constant2/1 -> Gain/1
  Matrix Exponential/1 -> Add/1, Divide2/1
  Divide2/1 -> mu Ts/1
  Add/1 -> Divide1/2
  x true/1 -> Add1/2
  Constant/1 -> Add/2
  Divide1/1 -> phi Ts/1
  Add1/1 -> Divide2/2  "x tilde"
  x hat/1 -> Add1/1
  Gain/1 -> Matrix Exponential/1

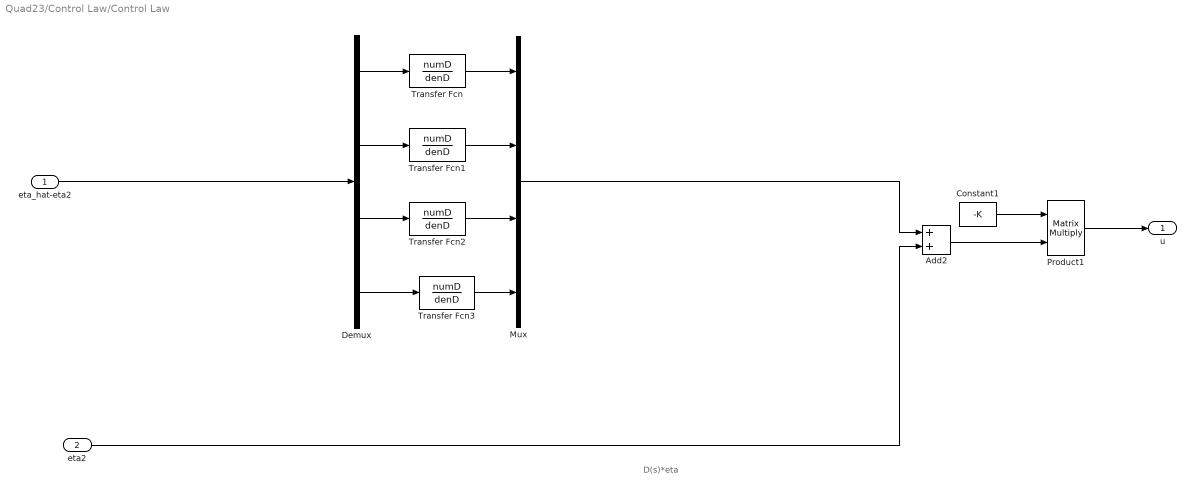
== system Quad23/Control Law/Control Law ==
  note: D(s)*eta
  eta_hat-eta2 : Inport
  eta2 : Inport  Port=2
  Add2 : Sum
  Constant1 : Constant  Value=-K
  Demux : Demux
  Mux : Mux
  Product1 : Product  Multiplication=Matrix(*)  RndMeth=Zero
  Transfer Fcn{,1..3} (4 alike) : TransferFcn  Numerator=numD  Denominator=denD
  u : Outport
  wires:
  Add2/1 -> Product1/2
  Constant1/1 -> Product1/1
  eta2/1 -> Add2/2
  Product1/1 -> u/1
  Mux/1 -> Add2/1
  eta_hat-eta2/1 -> Demux/1
  Demux/1 -> Transfer Fcn/1
  Transfer Fcn/1 -> Mux/1
  Demux/3 -> Transfer Fcn2/1
  Demux/2 -> Transfer Fcn1/1
  Transfer Fcn1/1 -> Mux/2
  Transfer Fcn2/1 -> Mux/3
  Demux/4 -> Transfer Fcn3/1
  Transfer Fcn3/1 -> Mux/4

== system Quad23/Control Law/Hm-1 Hum*D(s) ==
  sigma2 : Inport
  Add{,1..3} (4 alike) : Sum  Inputs=+++
  Demux : Demux  Outputs=3
  Mux : Mux
  Subsystem : Subsystem
  Subsystem1 : Subsystem
  Subsystem2 : Subsystem
  Subsystem3 : Subsystem
  eta2m : Outport
  wires:
  Mux/1 -> eta2m/1
  sigma2/1 -> Demux/1
  Add/1 -> Mux/1
  Subsystem/1(Out1) -> Add/1
  Subsystem/2(Out2) -> Add/2
  Subsystem/3(Out3) -> Add/3
  Add1/1 -> Mux/2
  Subsystem1/2(Out2) -> Add1/2
  Subsystem1/1(Out1) -> Add1/1
  Subsystem1/3(Out3) -> Add1/3
  Add2/1 -> Mux/3
  Subsystem2/2(Out2) -> Add2/2
  Subsystem2/1(Out1) -> Add2/1
  Subsystem2/3(Out3) -> Add2/3
  Subsystem3/3(Out3) -> Add3/3
  Subsystem3/1(Out1) -> Add3/1
  Subsystem3/2(Out2) -> Add3/2
  Add3/1 -> Mux/4
  Demux/1 -> Subsystem3/1(In1), Subsystem2/1(In1), Subsystem1/1(In1), Subsystem/1(In1)
  Demux/2 -> Subsystem3/2(In2), Subsystem2/2(In2), Subsystem1/2(In2), Subsystem/2(In2)
  Demux/3 -> Subsystem3/3(In3), Subsystem2/3(In3), Subsystem/3(In3), Subsystem1/3(In3)

== system Quad23/Control Law/Subsystem1 ==
  Forces and moment cmd : Inport
  Constant1 : Constant  Value=inv(LAMBDA)
  Only greater than zero : Subsystem
  Product : Product  Multiplication=Matrix(*)
  Sqrt : Sqrt  OutputSignalType=real  SaturateOnIntegerOverflow=on
  Engine speed cmd : Outport
  wires:
  Forces and moment cmd/1 -> Product/2
  Product/1 -> Only greater than zero/1(In1)
  Constant1/1 -> Product/1
  Sqrt/1 -> Engine speed cmd/1  "engine"
  Only greater than zero/1(Out1) -> Sqrt/1

== system Quad23/Control Law/eta hat computation ==
  u : Inport
  sigma1 : Inport  Port=2
  rg : Inport  Port=3
  Add : Sum  Inputs=++-
  Gain : Gain  Gain=omega0  Multiplication=Matrix(K*u)
  eta_hat-eta_2 : Outport
  wires:
  rg/1 -> Add/3
  u/1 -> Gain/1
  Gain/1 -> Add/1
  Add/1 -> eta_hat-eta_2/1
  sigma1/1 -> Add/2

== system Quad23/Control Law/state_feedback_NOMINAL ==
  Nominal FORCES MOMENT Request : Inport
  ENGINES : Subsystem  mask{LAMBDA=LAMBDA}
      mask prompts: LAMBDA "Insert Lambda Matrix"
  Square speeds : Subsystem
  Subsystem1 : Subsystem
  Out1 : Outport
  wires:
  Nominal FORCES MOMENT Request/1 -> Subsystem1/1(Forces and moment cmd)
  Square speeds/1(omega^2) -> ENGINES/1(OMEGA  SQUARE)
  Subsystem1/1(Engine speed cmd) -> Square speeds/1(Engine speed)
  ENGINES/1(GAMMA EFFECTS) -> Out1/1

== system Quad23/Control Law/u_ad_cmd2 u_ad_effect2 ==
  u adaptive : Inport
  ENGINES : Subsystem  mask{LAMBDA=LAMBDA}
      mask prompts: LAMBDA "Insert Lambda Matrix"
  Square speeds : Subsystem
  Subsystem1 : Subsystem
  Effect adaptive : Outport
  wires:
  u adaptive/1 -> Subsystem1/1(Forces and moment cmd)
  Square speeds/1(omega^2) -> ENGINES/1(OMEGA  SQUARE)
  Subsystem1/1(Engine speed cmd) -> Square speeds/1(Engine speed)
  ENGINES/1(GAMMA EFFECTS) -> Effect adaptive/1

== system Quad23/Equation of Motion/Subsystem ==
  ATTITUDE : Inport
  omega : Inport  Port=2
  FROM BODY2NED1 : MATLAB Function  TreatAsAtomicUnit=on
  Product1 : Product  Multiplication=Matrix(*)
  ATTITUDE DOT : Outport
  wires:
  ATTITUDE/1 -> FROM BODY2NED1/1(ATTITUDE)
  FROM BODY2NED1/1(MATRIX) -> Product1/1
  Product1/1 -> ATTITUDE DOT/1
  omega/1 -> Product1/2

== system Quad23/Equation of Motion/Subsystem1 ==
  ATTITUDE : Inport
  V : Inport  Port=2
  FROM BODY2NED : MATLAB Function  TreatAsAtomicUnit=on
  Product : Product  Multiplication=Matrix(*)
  POS DOT : Outport
  wires:
  FROM BODY2NED/1(DCM) -> Product/1
  Product/1 -> POS DOT/1
  ATTITUDE/1 -> FROM BODY2NED/1(ATTITUDE)
  V/1 -> Product/2

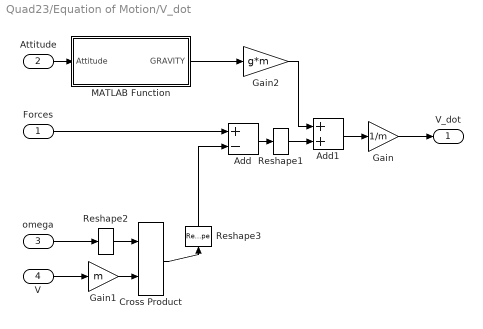
== system Quad23/Equation of Motion/V_dot  ==
  Forces : Inport
  Attitude : Inport  Port=2
  omega : Inport  Port=3
  V : Inport  Port=4
  Add : Sum  Inputs=+-
  Add1 : Sum
  Cross Product : vrlib/Utilities/Cross Product
      settings: SourceProductBaseCode=VR
  Gain : Gain  Gain=1/m
  Gain1 : Gain  Gain=m
  Gain2 : Gain  Gain=g*m
  MATLAB Function : MATLAB Function  TreatAsAtomicUnit=on
  Reshape1 : Reshape  OutputDimensionality=Column vector (2-D)
  Reshape2 : Reshape  OutputDimensionality=Column vector (2-D)
  Reshape3 : Reshape  OutputDimensionality=Column vector (2-D)
  V_dot : Outport
  wires:
  Forces/1 -> Add/1
  Add/1 -> Reshape1/1
  V/1 -> Gain1/1
  Cross Product/1 -> Reshape3/1
  Gain1/1 -> Cross Product/2
  Reshape2/1 -> Cross Product/1
  Reshape3/1 -> Add/2
  Add1/1 -> Gain/1
  Gain2/1 -> Add1/1
  Attitude/1 -> MATLAB Function/1(Attitude)
  MATLAB Function/1(GRAVITY) -> Gain2/1
  Gain/1 -> V_dot/1
  omega/1 -> Reshape2/1
  Reshape1/1 -> Add1/2

== system Quad23/Equation of Motion/omega dot ==
  omega : Inport
  Moment : Inport  Port=2
  Add : Sum  Inputs=+-
  Cross Product : vrlib/Utilities/Cross Product
      settings: SourceProductBaseCode=VR
  Gain1 : Gain  Gain=inertia  Multiplication=Matrix(K*u)
  Gain2 : Gain  Gain=inertia_inv  Multiplication=Matrix(K*u)
  omega_dot : Outport
  wires:
  Moment/1 -> Add/1
  Gain1/1 -> Cross Product/2
  omega/1 -> Cross Product/1, Gain1/1
  Cross Product/1 -> Add/2
  Add/1 -> Gain2/1
  Gain2/1 -> omega_dot/1

== system Quad23/Control Law/Hm-1 Hum*D(s)/Subsystem ==
  In1 : Inport
  In2 : Inport  Port=2
  In3 : Inport  Port=3
  Transfer Fcn : TransferFcn  Numerator=NUM_TF_eta2m_11  Denominator=DEN_TF_eta2m_11
  Transfer Fcn1 : TransferFcn  Numerator=NUM_TF_eta2m_13  Denominator=DEN_TF_eta2m_13
  Transfer Fcn3 : TransferFcn  Numerator=NUM_TF_eta2m_12  Denominator=DEN_TF_eta2m_12
  Out1 : Outport
  Out2 : Outport  Port=2
  Out3 : Outport  Port=3
  wires:
  In3/1 -> Transfer Fcn1/1
  In1/1 -> Transfer Fcn/1
  Transfer Fcn1/1 -> Out3/1
  Transfer Fcn/1 -> Out1/1
  In2/1 -> Transfer Fcn3/1
  Transfer Fcn3/1 -> Out2/1

== system Quad23/Control Law/Hm-1 Hum*D(s)/Subsystem1 ==
  In1 : Inport
  In2 : Inport  Port=2
  In3 : Inport  Port=3
  Transfer Fcn : TransferFcn  Numerator=NUM_TF_eta2m_21  Denominator=DEN_TF_eta2m_21
  Transfer Fcn1 : TransferFcn  Numerator=NUM_TF_eta2m_23  Denominator=DEN_TF_eta2m_23
  Transfer Fcn3 : TransferFcn  Numerator=NUM_TF_eta2m_22  Denominator=DEN_TF_eta2m_22
  Out1 : Outport
  Out2 : Outport  Port=2
  Out3 : Outport  Port=3
  wires:
  In3/1 -> Transfer Fcn1/1
  In1/1 -> Transfer Fcn/1
  Transfer Fcn1/1 -> Out3/1
  Transfer Fcn/1 -> Out1/1
  In2/1 -> Transfer Fcn3/1
  Transfer Fcn3/1 -> Out2/1

== system Quad23/Control Law/Hm-1 Hum*D(s)/Subsystem2 ==
  In1 : Inport
  In2 : Inport  Port=2
  In3 : Inport  Port=3
  Transfer Fcn : TransferFcn  Numerator=NUM_TF_eta2m_31  Denominator=DEN_TF_eta2m_31
  Transfer Fcn1 : TransferFcn  Numerator=NUM_TF_eta2m_33  Denominator=DEN_TF_eta2m_33
  Transfer Fcn3 : TransferFcn  Numerator=NUM_TF_eta2m_32  Denominator=DEN_TF_eta2m_32
  Out1 : Outport
  Out2 : Outport  Port=2
  Out3 : Outport  Port=3
  wires:
  In3/1 -> Transfer Fcn1/1
  In1/1 -> Transfer Fcn/1
  Transfer Fcn1/1 -> Out3/1
  Transfer Fcn/1 -> Out1/1
  In2/1 -> Transfer Fcn3/1
  Transfer Fcn3/1 -> Out2/1

== system Quad23/Control Law/Hm-1 Hum*D(s)/Subsystem3 ==
  In1 : Inport
  In2 : Inport  Port=2
  In3 : Inport  Port=3
  Transfer Fcn : TransferFcn  Numerator=NUM_TF_eta2m_41  Denominator=DEN_TF_eta2m_41
  Transfer Fcn1 : TransferFcn  Numerator=NUM_TF_eta2m_43  Denominator=DEN_TF_eta2m_43
  Transfer Fcn3 : TransferFcn  Numerator=NUM_TF_eta2m_42  Denominator=DEN_TF_eta2m_42
  Out1 : Outport
  Out2 : Outport  Port=2
  Out3 : Outport  Port=3
  wires:
  Transfer Fcn3/1 -> Out2/1
  In2/1 -> Transfer Fcn3/1
  Transfer Fcn/1 -> Out1/1
  Transfer Fcn1/1 -> Out3/1
  In1/1 -> Transfer Fcn/1
  In3/1 -> Transfer Fcn1/1

== system Quad23/Control Law/Subsystem1/Only greater than zero ==
  In1 : Inport
  Compare To Zero : simulink/Logic and Bit Operations/Compare To Zero  relop=>=  OutDataTypeStr=boolean
  Divide : Product  Inputs=**
  Out1 : Outport
  wires:
  In1/1 -> Compare To Zero/1, Divide/2
  Divide/1 -> Out1/1
  Compare To Zero/1 -> Divide/1

== system Quad23/Control Law/state_feedback_NOMINAL/ENGINES ==
  OMEGA  SQUARE : Inport
  Constant : Constant  Value=LAMBDA
  Product : Product  Multiplication=Matrix(*)
  GAMMA EFFECTS : Outport
  wires:
  Constant/1 -> Product/1
  Product/1 -> GAMMA EFFECTS/1
  OMEGA  SQUARE/1 -> Product/2

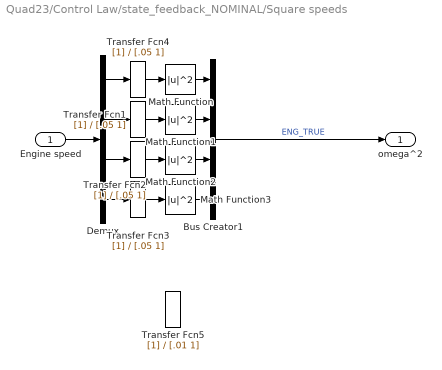
== system Quad23/Control Law/state_feedback_NOMINAL/Square speeds ==
  Engine speed : Inport
  Bus Creator1 : BusCreator  Inputs=4
  Demux : Demux
  Math Function{,1..3} (4 alike) : Math  Operator=magnitude^2  OutputSignalType=real  SaturateOnIntegerOverflow=on
  Transfer Fcn{1..4} (4 alike) : TransferFcn  Denominator=[.05 1]
  Transfer Fcn5 : TransferFcn  Denominator=[.01 1]
  omega^2 : Outport
  wires:
  Demux/4 -> Transfer Fcn3/1
  Demux/2 -> Transfer Fcn1/1
  Engine speed/1 -> Demux/1
  Demux/3 -> Transfer Fcn2/1
  Math Function3/1 -> Bus Creator1/4
  Math Function2/1 -> Bus Creator1/3
  Math Function1/1 -> Bus Creator1/2
  Math Function/1 -> Bus Creator1/1
  Demux/1 -> Transfer Fcn4/1
  Transfer Fcn4/1 -> Math Function/1
  Transfer Fcn1/1 -> Math Function1/1
  Transfer Fcn2/1 -> Math Function2/1
  Transfer Fcn3/1 -> Math Function3/1
  Bus Creator1/1 -> omega^2/1  "ENG_TRUE"

== system Quad23/Control Law/state_feedback_NOMINAL/Subsystem1 ==
  Forces and moment cmd : Inport
  Constant1 : Constant  Value=inv(LAMBDA)
  Only greater than zero : Subsystem
  Product : Product  Multiplication=Matrix(*)
  Sqrt : Sqrt  OutputSignalType=real  SaturateOnIntegerOverflow=on
  Engine speed cmd : Outport
  wires:
  Only greater than zero/1(Out1) -> Sqrt/1
  Sqrt/1 -> Engine speed cmd/1  "engine"
  Constant1/1 -> Product/1
  Product/1 -> Only greater than zero/1(In1)
  Forces and moment cmd/1 -> Product/2

== system Quad23/Control Law/u_ad_cmd2 u_ad_effect2/ENGINES ==
  OMEGA  SQUARE : Inport
  Constant : Constant  Value=LAMBDA
  Product : Product  Multiplication=Matrix(*)
  GAMMA EFFECTS : Outport
  wires:
  Constant/1 -> Product/1
  Product/1 -> GAMMA EFFECTS/1
  OMEGA  SQUARE/1 -> Product/2

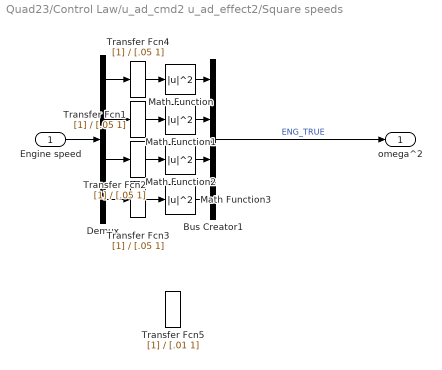
== system Quad23/Control Law/u_ad_cmd2 u_ad_effect2/Square speeds ==
  Engine speed : Inport
  Bus Creator1 : BusCreator  Inputs=4
  Demux : Demux
  Math Function{,1..3} (4 alike) : Math  Operator=magnitude^2  OutputSignalType=real  SaturateOnIntegerOverflow=on
  Transfer Fcn{1..4} (4 alike) : TransferFcn  Denominator=[.05 1]
  Transfer Fcn5 : TransferFcn  Denominator=[.01 1]
  omega^2 : Outport
  wires:
  Demux/4 -> Transfer Fcn3/1
  Demux/2 -> Transfer Fcn1/1
  Engine speed/1 -> Demux/1
  Demux/3 -> Transfer Fcn2/1
  Math Function3/1 -> Bus Creator1/4
  Math Function2/1 -> Bus Creator1/3
  Math Function1/1 -> Bus Creator1/2
  Math Function/1 -> Bus Creator1/1
  Demux/1 -> Transfer Fcn4/1
  Transfer Fcn4/1 -> Math Function/1
  Transfer Fcn1/1 -> Math Function1/1
  Transfer Fcn2/1 -> Math Function2/1
  Transfer Fcn3/1 -> Math Function3/1
  Bus Creator1/1 -> omega^2/1  "ENG_TRUE"

== system Quad23/Control Law/u_ad_cmd2 u_ad_effect2/Subsystem1 ==
  Forces and moment cmd : Inport
  Constant1 : Constant  Value=inv(LAMBDA)
  Only greater than zero : Subsystem
  Product : Product  Multiplication=Matrix(*)
  Sqrt : Sqrt  OutputSignalType=real  SaturateOnIntegerOverflow=on
  Engine speed cmd : Outport
  wires:
  Only greater than zero/1(Out1) -> Sqrt/1
  Sqrt/1 -> Engine speed cmd/1  "engine"
  Constant1/1 -> Product/1
  Product/1 -> Only greater than zero/1(In1)
  Forces and moment cmd/1 -> Product/2

== system Quad23/Control Law/state_feedback_NOMINAL/Subsystem1/Only greater than zero ==
  In1 : Inport
  Compare To Zero : simulink/Logic and Bit Operations/Compare To Zero  relop=>=  OutDataTypeStr=boolean
  Divide : Product  Inputs=**
  Out1 : Outport
  wires:
  Compare To Zero/1 -> Divide/1
  Divide/1 -> Out1/1
  In1/1 -> Divide/2, Compare To Zero/1

== system Quad23/Control Law/u_ad_cmd2 u_ad_effect2/Subsystem1/Only greater than zero ==
  In1 : Inport
  Compare To Zero : simulink/Logic and Bit Operations/Compare To Zero  relop=>=  OutDataTypeStr=boolean
  Divide : Product  Inputs=**
  Out1 : Outport
  wires:
  Compare To Zero/1 -> Divide/1
  Divide/1 -> Out1/1
  In1/1 -> Divide/2, Compare To Zero/1

== matlab function Quad23/Equation of Motion/Subsystem/FROM BODY2NED1 ==
  data: ATTITUDE input; MATRIX output
function MATRIX = MATRIX_PQR2ATTITUDE(ATTITUDE)

phi = ATTITUDE(1);
theta = ATTITUDE(2);
psi = ATTITUDE(3);
MATRIX = [1          0                 -sin(theta) 
         0        cos(phi)     sin(phi)*cos(theta)
         0       -sin(phi)     cos(theta)*cos(phi)];
end

== matlab function Quad23/Equation of Motion/Subsystem1/FROM BODY2NED ==
  data: ATTITUDE input; DCM output
function DCM = MATRIX(ATTITUDE)

phi = ATTITUDE(1);
theta = ATTITUDE(2);
psi = ATTITUDE(3);

DCM = [cos(psi)*cos(theta) cos(psi)*sin(theta)*sin(phi)-sin(psi)*cos(phi) cos(psi)*sin(theta)*cos(phi)+sin(psi)*sin(phi)
    sin(psi)*cos(theta) sin(psi)*sin(theta)*sin(phi)+cos(psi)*cos(phi) sin(psi)*sin(theta)*cos(phi)-cos(psi)*sin(phi)
    -sin(theta) cos(theta)*sin(phi) cos(theta)*cos(phi)];
end

== matlab function Quad23/Equation of Motion/V_dot /MATLAB Function ==
  data: Attitude input; GRAVITY output
function GRAVITY = GRAV(Attitude)

phi = Attitude(1);
theta = Attitude(2);
psi  = Attitude(3);

GRAVITY = [-sin(theta); cos(theta)*sin(phi); cos(theta)*cos(phi)];
end
